simulink model "IM_d_q"  (R2014a)
settings: Solver=ode3  SolverMode=SingleTasking  StartTime=0.0  StopTime=1  FixedStep=0.0001  RelTol=1e-3
values from neighbouring files (symbols this model uses):
  A1 = [-lamda ws ks/Tr 0; -ws -lamda 0 ks/Tr; M/Tr 0 -1/Tr ws; 0 M/Tr -ws -1/Tr;]    [IM_d_q.m]
  A2 = [0 0 0 ks; 0 0 -ks 0; 0 0 0 -1; 0 0 1 0]    [IM_d_q.m]
  B = [1/(Ls*sigma) 0; 0 1/(Ls*sigma); 0 0; 0 0]    [IM_d_q.m]
  f = 0    [IM_d_q.m]
  freq = 2*pi*50    (= 314.159265359)    [IM_d_q.m]
  J = 0.07    [IM_d_q.m]
  Lr = 0.1568    [IM_d_q.m]
  M = 0.15    [IM_d_q.m]
  p = 2    [IM_d_q.m]
  theta0 = 0    [IM_d_q.m]
  Vs = 200    [IM_d_q.m]
  ws = 2*pi*50    (= 314.159265359)    [IM_d_q.m]
settings Model: Creator=User  LastModifiedBy=User
settings DataIOCC: LimitDataPoints=off

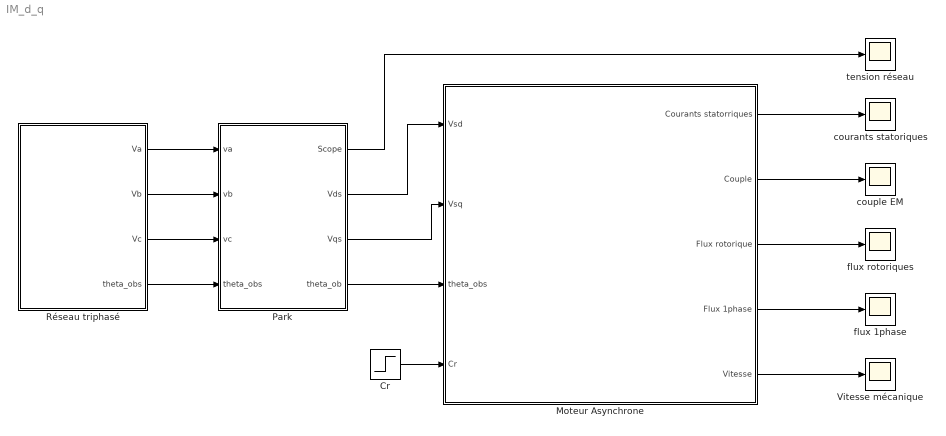
== system IM_d_q ==
  " courants statoriques" : Scope
      settings: SaveName=ScopeData8
  Cr : Step  After=15  SampleTime=0
  "Moteur Asynchrone " : Subsystem
  Park : Subsystem
  Réseau triphasé : Subsystem
  Vitesse mécanique : Scope
      settings: SaveName=ScopeData2
  couple EM : Scope
      settings: SaveName=ScopeData3
  flux 1phase : Scope
      settings: SaveName=ScopeData5
  flux rotoriques : Scope
      settings: SaveName=ScopeData4
  tension réseau : Scope
  wires:
  Réseau triphasé/1(Va) -> Park/1(va)
  Réseau triphasé/2(Vb) -> Park/2(vb)
  Réseau triphasé/3(Vc) -> Park/3(vc)
  Réseau triphasé/4(theta_obs) -> Park/4(theta_obs)
  Park/1(Scope) -> tension réseau/1
  Park/2(Vds) -> "Moteur Asynchrone "/1(Vsd)
  Park/3(Vqs) -> "Moteur Asynchrone "/2(Vsq)
  "Moteur Asynchrone "/1(Courants statorriques) -> " courants statoriques"/1
  "Moteur Asynchrone "/2(Couple) -> couple EM/1
  "Moteur Asynchrone "/3(Flux rotorique) -> flux rotoriques/1
  "Moteur Asynchrone "/4(Flux 1phase) -> flux 1phase/1
  "Moteur Asynchrone "/5(Vitesse) -> Vitesse mécanique/1
  Park/4(theta_ob) -> "Moteur Asynchrone "/3(theta_obs)
  Cr/1 -> "Moteur Asynchrone "/4(Cr)

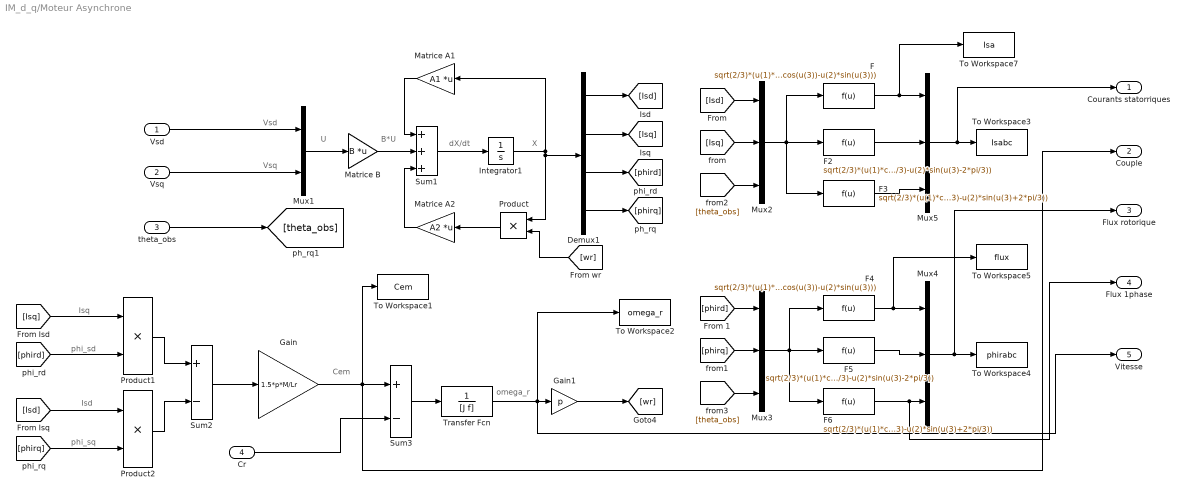
== system IM_d_q/Moteur Asynchrone  ==
  note: Cem
  note: omega_r
  note: Isd
  note: phi_sq
  note: phi_sd
  note: Isq
  note: dX/dt
  note: B*U
  note: U
  note: Vsq
  note: Vsd
  note: X
  Vsd : Inport
  Vsq : Inport  Port=2
  theta_obs : Inport  Port=3
  Cr : Inport  Port=4
  Demux1 : Demux
  F : Fcn  Expr=sqrt(2/3)*(u(1)*cos(u(3))-u(2)*sin(u(3)))
  F2 : Fcn  Expr=sqrt(2/3)*(u(1)*cos(u(3)-2*pi/3)-u(2)*sin(u(3)-2*pi/3))
  F3 : Fcn  Expr=sqrt(2/3)*(u(1)*cos(u(3)+2*pi/3)-u(2)*sin(u(3)+2*pi/3))
  F4 : Fcn  Expr=sqrt(2/3)*(u(1)*cos(u(3))-u(2)*sin(u(3)))
  F5 : Fcn  Expr=sqrt(2/3)*(u(1)*cos(u(3)-2*pi/3)-u(2)*sin(u(3)-2*pi/3))
  F6 : Fcn  Expr=sqrt(2/3)*(u(1)*cos(u(3)+2*pi/3)-u(2)*sin(u(3)+2*pi/3))
  Gain : Gain  Gain=1.5*p*M/Lr
  Gain1 : Gain  Gain=p
  Integrator1 : Integrator
  Matrice A1 : Gain  Gain=A1  Multiplication=Matrix(K*u)
  Matrice A2 : Gain  Gain=A2  Multiplication=Matrix(K*u)
  Matrice B : Gain  Gain=B  Multiplication=Matrix(K*u)
  Mux1 : Mux  Inputs=2
  Mux{2..5} (4 alike) : Mux  Inputs=3
  Product : Product
  Product1 : Product
  Product2 : Product
  Sum1 : Sum  Inputs=+++
  Sum2 : Sum  Inputs=+-
  Sum3 : Sum  Inputs=+-
  To Workspace1 : ToWorkspace  VariableName=Cem  SaveFormat=Timeseries  SampleTime=-1
  To Workspace2 : ToWorkspace  VariableName=omega_r  SaveFormat=Timeseries  SampleTime=-1
  To Workspace3 : ToWorkspace  VariableName=Isabc  SaveFormat=Timeseries  SampleTime=-1
  To Workspace4 : ToWorkspace  VariableName=phirabc  SaveFormat=Timeseries  SampleTime=-1
  To Workspace5 : ToWorkspace  VariableName=flux  SaveFormat=Timeseries  SampleTime=-1
  To Workspace7 : ToWorkspace  VariableName=Isa  SaveFormat=Timeseries  SampleTime=-1
  Transfer Fcn : TransferFcn  Denominator=[J f]
  Courants statorriques : Outport
  Couple : Outport  Port=2
  Flux rotorique : Outport  Port=3
  Flux 1phase : Outport  Port=4
  Vitesse : Outport  Port=5
  wires:
  Vsq/1 -> Mux1/2
  Vsd/1 -> Mux1/1
  Product/1 -> Matrice A2/1
  Matrice A1/1 -> Sum1/1
  Matrice A2/1 -> Sum1/3
  F/1 -> To Workspace7/1, Mux5/1
  Mux3/1 -> F6/1, F4/1, F5/1
  F5/1 -> Mux4/2
  F6/1 -> Flux 1phase/1, Mux4/3
  [wr] -> Product/2
  Demux1/1 -> [Isd]
  Product1/1 -> Sum2/1
  Demux1/4 -> [phirq]
  Gain1/1 -> [wr]
  [Isq] -> Product1/1
  F3/1 -> Mux5/3
  Product2/1 -> Sum2/2
  Cr/1 -> Sum3/2
  Matrice B/1 -> Sum1/2
  Mux1/1 -> Matrice B/1
  Sum2/1 -> Gain/1
  Sum3/1 -> Transfer Fcn/1
  Integrator1/1 -> Matrice A1/1, Product/1, Demux1/1
  Demux1/3 -> [phird]
  Sum1/1 -> Integrator1/1
  [phird] -> Product1/2
  [phird] -> Mux3/1
  [Isq] -> Mux2/2
  [phirq] -> Mux3/2
  [phirq] -> Product2/2
  Gain/1 -> Couple/1, To Workspace1/1, Sum3/1
  Demux1/2 -> [Isq]
  [Isd] -> Product2/1
  [Isd] -> Mux2/1
  F2/1 -> Mux5/2
  [theta_obs] -> Mux2/3
  F4/1 -> To Workspace5/1, Mux4/1
  Mux4/1 -> Flux rotorique/1, To Workspace4/1
  Mux2/1 -> F/1, F3/1, F2/1
  Transfer Fcn/1 -> Vitesse/1, To Workspace2/1, Gain1/1
  [theta_obs] -> Mux3/3
  Mux5/1 -> Courants statorriques/1, To Workspace3/1
  theta_obs/1 -> [theta_obs]

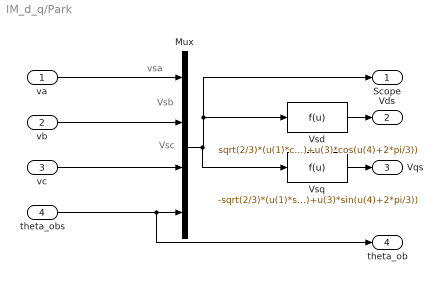
== system IM_d_q/Park ==
  note: Vsc
  note: Vsb
  note: vsa
  va : Inport
  vb : Inport  Port=2
  vc : Inport  Port=3
  theta_obs : Inport  Port=4
  Mux : Mux
  Vsd : Fcn  Expr=sqrt(2/3)*(u(1)*cos(u(4))+u(2)*cos(u(4)-2*pi/3)+u(3)*cos(u(4)+2*pi/3))
  Vsq : Fcn  Expr=-sqrt(2/3)*(u(1)*sin(u(4))+u(2)*sin(u(4)-2*pi/3)+u(3)*sin(u(4)+2*pi/3))
  Scope : Outport
  Vds : Outport  Port=2
  Vqs : Outport  Port=3
  theta_ob : Outport  Port=4
  wires:
  Vsd/1 -> Vds/1
  Vsq/1 -> Vqs/1
  theta_obs/1 -> theta_ob/1, Mux/4
  va/1 -> Mux/1
  vb/1 -> Mux/2
  vc/1 -> Mux/3
  Mux/1 -> Vsq/1, Scope/1, Vsd/1

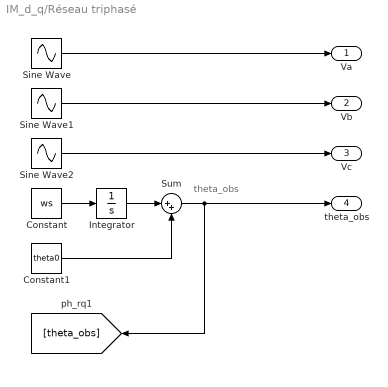
== system IM_d_q/Réseau triphasé ==
  note: theta_obs
  Constant : Constant  Value=ws
  Constant1 : Constant  Value=theta0
  Integrator : Integrator
  Sine Wave : Sin  Amplitude=Vs  Frequency=freq  SampleTime=0
  Sine Wave1 : Sin  Amplitude=Vs  Frequency=freq  Phase=-2*pi/3  SampleTime=0
  Sine Wave2 : Sin  Amplitude=Vs  Frequency=freq  Phase=2*pi/3  SampleTime=0
  Sum : Sum  Inputs=|++
  Va : Outport
  Vb : Outport  Port=2
  Vc : Outport  Port=3
  theta_obs : Outport  Port=4
  wires:
  Constant1/1 -> Sum/2
  Sine Wave1/1 -> Vb/1
  Constant/1 -> Integrator/1
  Sine Wave/1 -> Va/1
  Sine Wave2/1 -> Vc/1
  Integrator/1 -> Sum/1
  Sum/1 -> theta_obs/1, [theta_obs]
